simulink library "Electrical_Vehicle_Data_Calculation"  (R2017b)
settings: Solver=VariableStepAuto  StartTime=0.0  StopTime=10.0  RelTol=1e-3
undefined symbols (not defined in the file): DiscIntNeverNeededParam
settings Model: Creator=Alexander Koch  LastModifiedBy=ga69qig
settings CodeAppCC: StateflowObjectComments=on

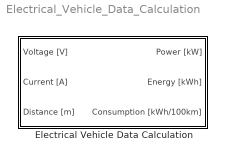
== system Electrical_Vehicle_Data_Calculation ==
  Electrical Vehicle Data Calculation : Subsystem

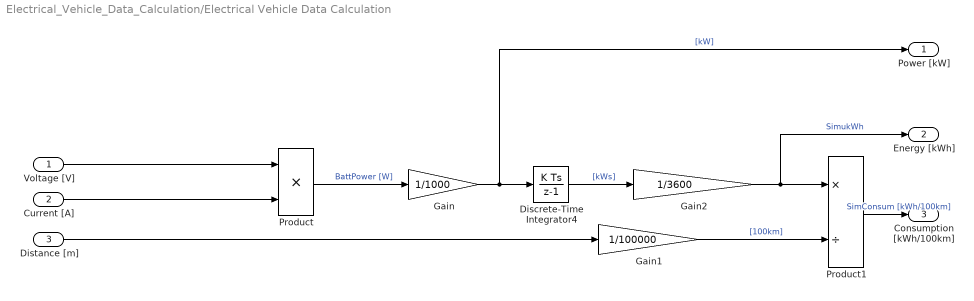
== system Electrical_Vehicle_Data_Calculation/Electrical Vehicle Data Calculation ==
  Voltage [V] : Inport
  Current [A] : Inport  Port=2
  Distance [m] : Inport  Port=3
  Discrete-Time Integrator4 : DiscreteIntegrator  InitialConditionSetting=State (most efficient)  SampleTime=-1  ICPrevOutput=DiscIntNeverNeededParam  ICPrevScaledInput=DiscIntNeverNeededParam
  Gain : Gain  Gain=1/1000
  Gain1 : Gain  Gain=1/100000
  Gain2 : Gain  Gain=1/3600
  Product : Product
  Product1 : Product  Inputs=*/
  Power [kW] : Outport
  Energy [kWh] : Outport  Port=2
  Consumption [kWh/100km] : Outport  Port=3
  wires:
  Voltage [V]/1 -> Product/1
  Product/1 -> Gain/1  "BattPower [W]"
  Gain/1 -> Power [kW]/1, Discrete-Time Integrator4/1  "[kW]"
  Discrete-Time Integrator4/1 -> Gain2/1  "[kWs]"
  Gain1/1 -> Product1/2  "[100km]"
  Product1/1 -> Consumption [kWh/100km]/1  "SimConsum [kWh/100km]"
  Current [A]/1 -> Product/2
  Gain2/1 -> Energy [kWh]/1, Product1/1  "SimukWh"
  Distance [m]/1 -> Gain1/1
